simulink model "Loops8"  (Simulink 6.0)
settings: Solver=ode45  StartTime=0.0  StopTime=10.0  RelTol=1e-3
settings Model: Creator=scaife  LastModifiedBy=scaife  ExtModeAutoUpdateStatusClock=off
settings DataIOCC: SignalLoggingName=sigsOut
settings DebuggingCC: SolverPrmCheckMsg=none
settings HardwareCC: TargetUnknown=on
settings GRTTargetCC: ModelReferenceCompliant=off  MatFileLogging=off

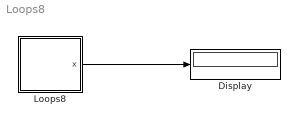
== system Loops8 ==
  Display : Display
  Loops8 : Stateflow chart
  wires:
  Loops8/1(x) -> Display/1

== stateflow chart Loops8 ==
  state A
  state B
  state C
  state D
  (default) -> A
  (junction 8) -> B : [x==0]
  (junction 10) -> D : [x==2]
  A -> (junction 9) : {x=0}
  C -> (junction 7) : {x=2}
  (junction 9) -> (junction 7) : [x==0]
  (junction 7) -> (junction 9) : [x==2]
  (junction 8) -> (junction 9) : [x==3]
  (junction 9) -> (junction 8) : [x==2]
  (junction 8) -> (junction 10) : [x==1||x==2]
  (junction 10) -> (junction 8) : [x==0||x==3]
  (junction 7) -> (junction 10) : [x==0]
  (junction 10) -> (junction 7) : [x==1]
  B -> (junction 8) : {x=1}
  D -> (junction 10) : {x=3}
  (junction 7) -> C : [x==1]
  (junction 9) -> A : [x==3]
  data: x output int32
